simulink library "INT_ErrLmp_DD"  (R2016b)
settings: Solver=VariableStepAuto  StartTime=0.0  StopTime=10.0  RelTol=1e-3
settings Model: Creator=liutao  LastModifiedBy=liutao

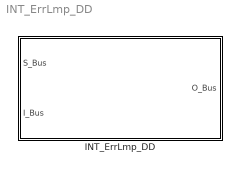
== system INT_ErrLmp_DD ==
  INT_ErrLmp_DD : Subsystem

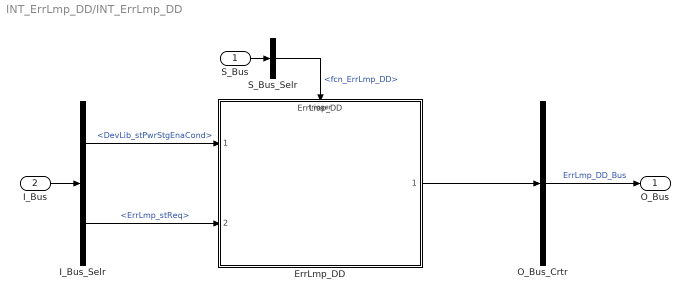
== system INT_ErrLmp_DD/INT_ErrLmp_DD ==
  S_Bus : Inport
  I_Bus : Inport  Port=2
  ErrLmp_DD : ModelReference  ModelNameDialog=ErrLmp_DD  SimulationMode=Normal  ModelReferenceVersion=1.9  TriggerPortName=function  TriggerPortTriggerType=function-call  TriggerPortStatesWhenEnabling=held
  I_Bus_Selr : BusSelector  OutputSignals=DevLib_stPwrStgEnaCond,ErrLmp_stReq
  O_Bus_Crtr : BusCreator  Inputs=1
  S_Bus_Selr : BusSelector  OutputSignals=fcn_ErrLmp_DD
  O_Bus : Outport
  wires:
  S_Bus_Selr/1 -> ErrLmp_DD/Trigger  "<fcn_ErrLmp_DD>"
  S_Bus/1 -> S_Bus_Selr/1
  I_Bus/1 -> I_Bus_Selr/1
  I_Bus_Selr/1 -> ErrLmp_DD/1  "<DevLib_stPwrStgEnaCond>"
  I_Bus_Selr/2 -> ErrLmp_DD/2  "<ErrLmp_stReq>"
  O_Bus_Crtr/1 -> O_Bus/1  "ErrLmp_DD_Bus"
  ErrLmp_DD/1 -> O_Bus_Crtr/1
